simulink model "dc_series_motor_performance"  (R2017a)
settings: Solver=VariableStepAuto  StartTime=0.0  StopTime=0.6  RelTol=1e-3
settings Model: Creator=Md Aadil  LastModifiedBy=Md Aadil

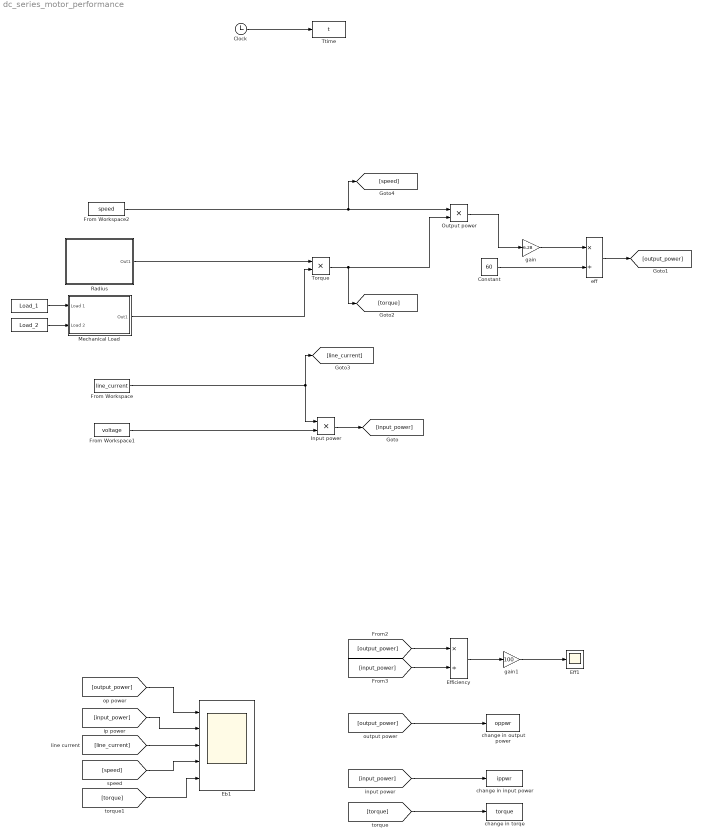
== system dc_series_motor_performance ==
  " " : FromWorkspace  VariableName=Load_1
  "  " : FromWorkspace  VariableName=Load_2
  Clock : Clock
  Constant : Constant  Value=60
  Eb1 : Scope  NumInputPorts=5
  "Eff1 " : Scope
  "Efficiency " : Product  Inputs=*/
  From Workspace : FromWorkspace  VariableName=line_current  SampleTime=0.1
  From Workspace1 : FromWorkspace  VariableName=voltage
  From Workspace2 : FromWorkspace  VariableName=speed
  Input power : Product
  Mechanical Load : Subsystem
  Output power : Product
  Radius : Subsystem
  Torque : Product
  Ttime : ToWorkspace  VariableName=t  SampleTime=-1
  "change in input power " : ToWorkspace  VariableName=ippwr  SampleTime=-1
  change in output power : ToWorkspace  VariableName=oppwr  SampleTime=-1
  change in torqe : ToWorkspace  VariableName=torque  SampleTime=-1
  eff : Product  Inputs=*/
  gain : Gain  Gain=6.28
  gain1 : Gain  Gain=100
  wires:
  [line_current] -> Eb1/3
  [output_power] -> "Efficiency "/1
  [output_power] -> Eb1/1
  [torque] -> change in torqe/1
  [speed] -> Eb1/4
  From Workspace/1 -> [line_current], Input power/1
  [output_power] -> change in output power/1
  From Workspace2/1 -> [speed], Output power/1
  "  "/1 -> Mechanical Load/2(Load 2)
  Torque/1 -> [torque], Output power/2
  [input_power] -> "Efficiency "/2
  From Workspace1/1 -> Input power/2
  Radius/1(Out1) -> Torque/1
  [input_power] -> Eb1/2
  [input_power] -> "change in input power "/1
  Mechanical Load/1(Out1) -> Torque/2
  Clock/1 -> Ttime/1
  Input power/1 -> [input_power]
  " "/1 -> Mechanical Load/1(Load 1)
  [torque] -> Eb1/5
  Constant/1 -> eff/2
  eff/1 -> [output_power]
  gain/1 -> eff/1
  Output power/1 -> gain/1
  "Efficiency "/1 -> gain1/1
  gain1/1 -> "Eff1 "/1

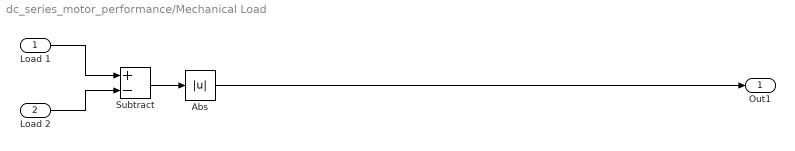
== system dc_series_motor_performance/Mechanical Load ==
  Load 1 : Inport
  Load 2 : Inport  Port=2
  Abs : Abs
  Subtract : Sum  Inputs=+-
  Out1 : Outport
  wires:
  Load 1/1 -> Subtract/1
  Load 2/1 -> Subtract/2
  Abs/1 -> Out1/1
  Subtract/1 -> Abs/1

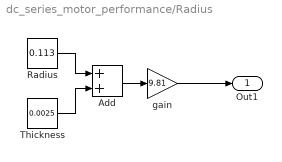
== system dc_series_motor_performance/Radius ==
  Add : Sum
  Radius : Constant  Value=0.113
  Thickness : Constant  Value=0.0025
  gain : Gain  Gain=9.81
  Out1 : Outport
  wires:
  Radius/1 -> Add/1
  Thickness/1 -> Add/2
  Add/1 -> gain/1
  gain/1 -> Out1/1
